simulink model "BPM_VA_Spin_Variants"  (R2022b)
settings: Solver=FixedStepDiscrete  StartTime=0.0  StopTime=10.0  FixedStep=TimeSteps.ModelStep  RelTol=1e-3
settings Model: Creator=KIRTACA  LastModifiedBy=BEDNASA
settings SolverCC: AlgebraicLoopSolver=TrustRegion
settings DataIOCC: ReturnWorkspaceOutputs=off
settings DebuggingCC: UnconnectedInputMsg=warning  UnconnectedOutputMsg=warning  UnconnectedLineMsg=warning  SFMachineParentedDataDiag=warning  ArithmeticOperatorsInVariantConditions=warning
settings ModelReferenceCC: EnableRefExpFcnMdlSchedulingChecks=on
settings SFSimCC: SimUseLocalCustomCode=off  CustomCodeUndefinedFunction=UseInterfaceOnly
settings RTWCC: RTWUseLocalCustomCode=off  RTWUseSimCustomCode=on
settings CodeAppCC: StateflowObjectComments=on

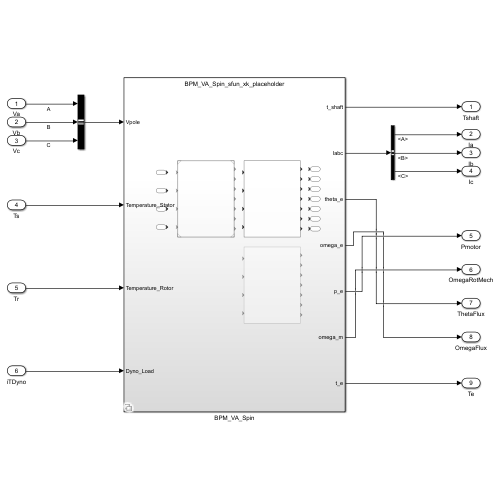
[thumbnail: Simulink's stored preview of the top-level diagram]
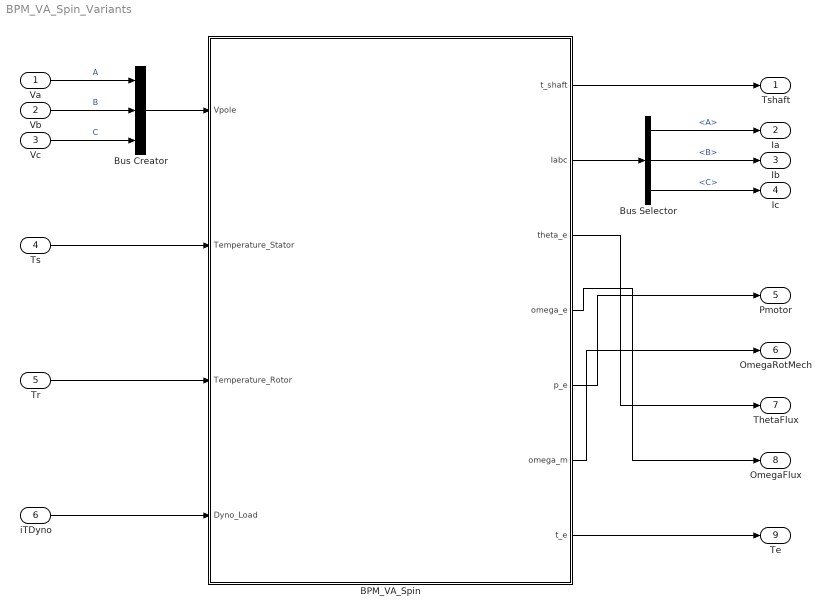
== system BPM_VA_Spin_Variants ==
  Va : Inport
  Vb : Inport  Port=2
  Vc : Inport  Port=3
  Ts : Inport  Port=4
  Tr : Inport  Port=5
  iTDyno : Inport  Port=6
  BPM_VA_Spin : Subsystem  Variant=on  VariantControl=Variant1
  Bus Creator : BusCreator  Inputs=3
  Bus Selector : BusSelector  OutputSignals=A,B,C
  Tshaft : Outport  VectorParamsAs1DForOutWhenUnconnected=off
  Ia : Outport  Port=2  VectorParamsAs1DForOutWhenUnconnected=off
  Ib : Outport  Port=3  VectorParamsAs1DForOutWhenUnconnected=off
  Ic : Outport  Port=4  VectorParamsAs1DForOutWhenUnconnected=off
  Pmotor : Outport  Port=5  VectorParamsAs1DForOutWhenUnconnected=off
  OmegaRotMech : Outport  Port=6  VectorParamsAs1DForOutWhenUnconnected=off
  ThetaFlux : Outport  Port=7  VectorParamsAs1DForOutWhenUnconnected=off
  OmegaFlux : Outport  Port=8  VectorParamsAs1DForOutWhenUnconnected=off
  Te : Outport  Port=9  VectorParamsAs1DForOutWhenUnconnected=off
  wires:
  Bus Selector/2 -> Ib/1  "<B>"
  Bus Selector/1 -> Ia/1  "<A>"
  BPM_VA_Spin/5(p_e) -> Pmotor/1
  BPM_VA_Spin/1(t_shaft) -> Tshaft/1
  BPM_VA_Spin/6(omega_m) -> OmegaRotMech/1
  BPM_VA_Spin/3(theta_e) -> ThetaFlux/1
  BPM_VA_Spin/2(Iabc) -> Bus Selector/1
  BPM_VA_Spin/4(omega_e) -> OmegaFlux/1
  Bus Selector/3 -> Ic/1  "<C>"
  BPM_VA_Spin/7(t_e) -> Te/1
  Vb/1 -> Bus Creator/2  "B"
  iTDyno/1 -> BPM_VA_Spin/4(Dyno_Load)
  Ts/1 -> BPM_VA_Spin/2(Temperature_Stator)
  Bus Creator/1 -> BPM_VA_Spin/1(Vpole)
  Vc/1 -> Bus Creator/3  "C"
  Va/1 -> Bus Creator/1  "A"
  Tr/1 -> BPM_VA_Spin/3(Temperature_Rotor)

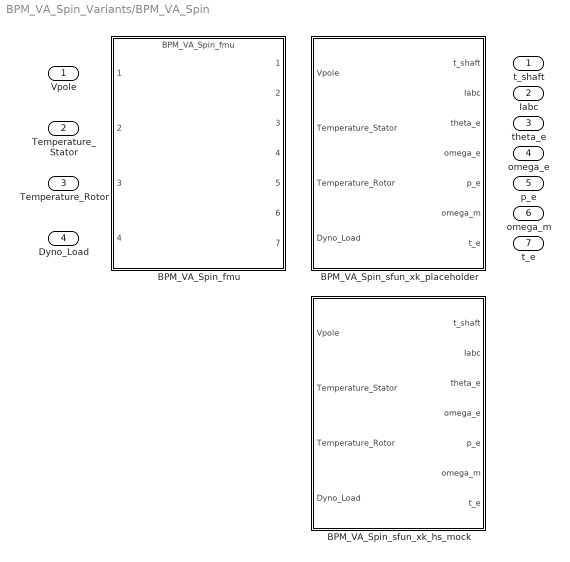
== system BPM_VA_Spin_Variants/BPM_VA_Spin ==
  Vpole : Inport  OutDataTypeStr=Bus: XabcBus
  Temperature_Stator : Inport  Port=2
  Temperature_Rotor : Inport  Port=3
  Dyno_Load : Inport  Port=4
  BPM_VA_Spin_fmu : ModelReference  ModelNameDialog=BPM_VA_Spin_fmu.slx  UsingDefaultArgumentValue=0,0,0,0,0,0,0,0,0,0,0,0,0,0,0,0,0,0,0,0,0,0,0,0,0,0,0,0,0,0,0,0,0,0,0,0,0,0,0,0,0,0,0,0,0,0,0,0,0,0,0  SimulationMode=Normal  VariantControl=Variant_Motor_Model_Executable == 1  ModelReferenceVersion=10.11  bpm_Rs_0=Motor_prm.Electrical.Rs_0  bpm_Ld_0=Motor_prm.Electrical.Ld_0  bpm_Lq_0=Motor_prm.Electrical.Lq_0  bpm_PM_flux_h1_0=Motor_prm.Electrical.PM_flux_h1_0  bpm_NPP=Motor_prm.Electrical.NPP  bpm_Jrotor=Motor_prm.Mechanical.Jrotor  bpm_B=Motor_prm.Mechanical.B  bpm_TR=Motor_prm.Mechanical.TR  bpm_Temp_stator_0=Motor_prm.Thermal.Temp_stator_0  bpm_Temp_rotor_0=Motor_prm.Thermal.Temp_rotor_0  bpm_Rs_stator_alpha=Motor_prm.Thermal.Rs_alpha  bpm_PM_rotor_alpha=Motor_prm.Thermal.PM_alpha  bpm_Ls_sat_flag=1  bpm_Loss_flag=Motor_prm.Power_Loss.Flag  bpm_Loss_th=10  bpm_Rsa_aux=0  bpm_Rsb_aux=0  bpm_Rsc_aux=0  Mech_HAs_J_drum=0  Mech_HAs_damp=0  Mech_HAs_m_unb=0  Mech_HAs_r_unb=0  Mech_HAs_TR=0  Mech_HAs_CF=0  Mech_VAa_water_vol=0  Mech_VAa_imp_dens=0  Mech_VAa_gear_ratio=0  Mech_VAa_clothes_mass=0  Mech_VAa_belt_ratio=0  Mech_VAa_basket_dia=0  Mech_VAa_basket_dens=0  Mech_VAa_J_basket=0  Mech_VAa_J_impeller=0  Mech_VAs_m_u=Mechanical.m_u  Mech_VAs_m_t=Mechanical.m_t  Mech_VAs_m_d=Mechanical.m_d  Mech_VAs_m_b1=Mechanical.m_b1  Mech_VAs_m_b2=Mechanical.m_b2  Mech_VAs_e=Mechanical.e  Mech_VAs_d=Mechanical.d  Mech_VAs_belt_rat=Mechanical.belt_ratio  Mech_VAs_T_f=Mechanical.T_f  Mech_VAs_K=2700  Mech_VAs_I_zt=Mechanical.I_zt  Mech_VAs_D_r=Mechanical.D_r  SimulationMode=Normal
  BPM_VA_Spin_sfun_xk_hs_mock : Subsystem  VariantControl=Variant_Motor_Model_Executable == 21
  BPM_VA_Spin_sfun_xk_placeholder : Subsystem  VariantControl=Variant_Motor_Model_Executable == 2
  t_shaft : Outport  VectorParamsAs1DForOutWhenUnconnected=off
  Iabc : Outport  Port=2  OutDataTypeStr=Bus: XabcBus  VectorParamsAs1DForOutWhenUnconnected=off
  theta_e : Outport  Port=3  VectorParamsAs1DForOutWhenUnconnected=off
  omega_e : Outport  Port=4  VectorParamsAs1DForOutWhenUnconnected=off
  p_e : Outport  Port=5  VectorParamsAs1DForOutWhenUnconnected=off
  omega_m : Outport  Port=6  VectorParamsAs1DForOutWhenUnconnected=off
  t_e : Outport  Port=7  VectorParamsAs1DForOutWhenUnconnected=off

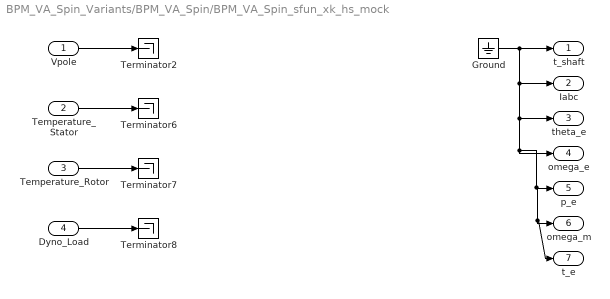
== system BPM_VA_Spin_Variants/BPM_VA_Spin/BPM_VA_Spin_sfun_xk_hs_mock ==
  Vpole : Inport  OutDataTypeStr=Bus: XabcBus
  Temperature_Stator : Inport  Port=2
  Temperature_Rotor : Inport  Port=3
  Dyno_Load : Inport  Port=4
  Ground : Ground
  Terminator{2,6..8} (4 alike) : Terminator
  t_shaft : Outport  VectorParamsAs1DForOutWhenUnconnected=off
  Iabc : Outport  Port=2  OutDataTypeStr=Bus: XabcBus  VectorParamsAs1DForOutWhenUnconnected=off
  theta_e : Outport  Port=3  VectorParamsAs1DForOutWhenUnconnected=off
  omega_e : Outport  Port=4  VectorParamsAs1DForOutWhenUnconnected=off
  p_e : Outport  Port=5  VectorParamsAs1DForOutWhenUnconnected=off
  omega_m : Outport  Port=6  VectorParamsAs1DForOutWhenUnconnected=off
  t_e : Outport  Port=7  VectorParamsAs1DForOutWhenUnconnected=off
  wires:
  Vpole/1 -> Terminator2/1
  Temperature_Stator/1 -> Terminator6/1
  Temperature_Rotor/1 -> Terminator7/1
  Dyno_Load/1 -> Terminator8/1
  Ground/1 -> t_e/1, omega_m/1, p_e/1, omega_e/1, theta_e/1, Iabc/1, t_shaft/1

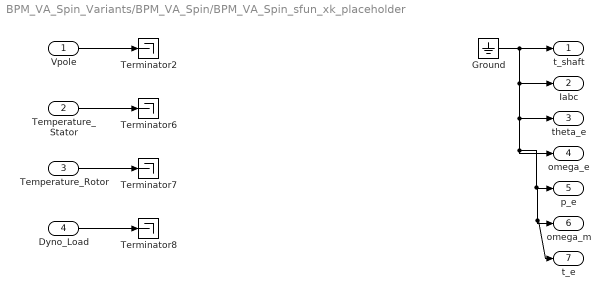
== system BPM_VA_Spin_Variants/BPM_VA_Spin/BPM_VA_Spin_sfun_xk_placeholder ==
  Vpole : Inport  OutDataTypeStr=Bus: XabcBus
  Temperature_Stator : Inport  Port=2
  Temperature_Rotor : Inport  Port=3
  Dyno_Load : Inport  Port=4
  Ground : Ground
  Terminator{2,6..8} (4 alike) : Terminator
  t_shaft : Outport  VectorParamsAs1DForOutWhenUnconnected=off
  Iabc : Outport  Port=2  OutDataTypeStr=Bus: XabcBus  VectorParamsAs1DForOutWhenUnconnected=off
  theta_e : Outport  Port=3  VectorParamsAs1DForOutWhenUnconnected=off
  omega_e : Outport  Port=4  VectorParamsAs1DForOutWhenUnconnected=off
  p_e : Outport  Port=5  VectorParamsAs1DForOutWhenUnconnected=off
  omega_m : Outport  Port=6  VectorParamsAs1DForOutWhenUnconnected=off
  t_e : Outport  Port=7  VectorParamsAs1DForOutWhenUnconnected=off
  wires:
  Vpole/1 -> Terminator2/1
  Temperature_Stator/1 -> Terminator6/1
  Temperature_Rotor/1 -> Terminator7/1
  Dyno_Load/1 -> Terminator8/1
  Ground/1 -> t_e/1, omega_m/1, p_e/1, omega_e/1, theta_e/1, Iabc/1, t_shaft/1
